simulink model "waypointFollower_Kohei"  (R2025a)
settings: Solver=ode23tb  StartTime=0.0  StopTime=130  FixedStep=.005  RelTol=1e-3  EnableMultiTasking=on
undefined symbols (not defined in the file): Cd, DiscIntNeverNeededParam, Kd_alt, Kd_p, Kd_q, Ki_alt, Ki_yaw, Kp_alt, Kp_p, Kp_pitch, Kp_pos, Kp_q, Kp_r, Kp_roll, Kp_vel, Kp_yaw, mass, mission, N_alt, N_p, N_q, rotorDir, rotorPositions, rotorThrustMax, rotorTimeConst, rotorTorqueMax, UAVsampleTime, x_area, y_area, z_area
libraries: simulink x9, slpidlib x9, uavalgslib x2, sim3dlib x2, uavsim3dlib x2, aerolibatmos2 x1, aerolibwind2 x1, shared6dof x1
(part 2 of 2)

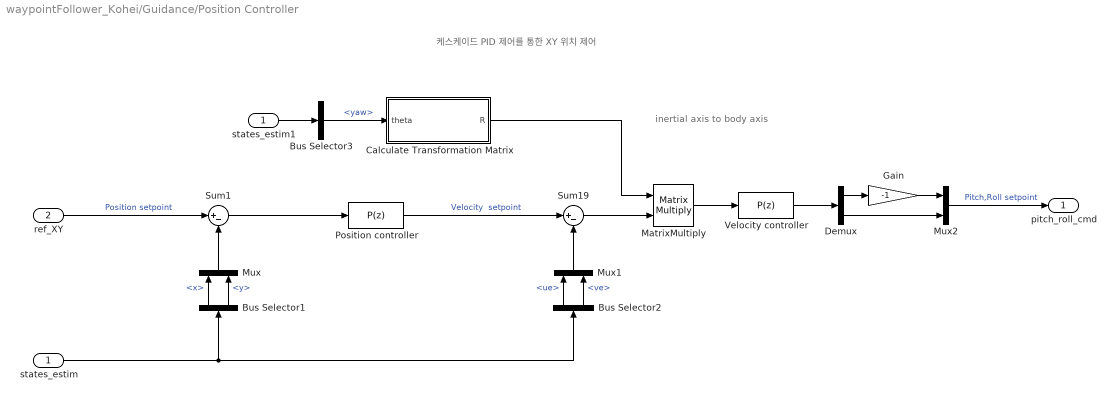
== system waypointFollower_Kohei/Guidance/Position Controller ==
  note: 케스케이드 PID 제어를 통한 XY 위치 제어
  note: inertial axis to body axis
  states_estim : Inport  OutDataTypeStr=Bus: UAVStateBUS
  ref_XY : Inport  Port=2
  Bus Selector1 : BusSelector  OutputSignals=x,y
  Bus Selector2 : BusSelector  OutputSignals=ue,ve
  Bus Selector3 : BusSelector  OutputSignals=yaw
  Calculate Transformation Matrix : Subsystem
  Demux : Demux  Outputs=2
  Gain : Gain  Gain=-1
  MatrixMultiply : Product  Multiplication=Matrix(*)
  Mux : Mux  Inputs=2
  Mux1 : Mux  Inputs=2
  Mux2 : Mux  Inputs=2
  Position controller : slpidlib/PID Controller  Controller=P  Form=Parallel  TimeDomain=Discrete-time  UseExternalTs=off  SampleTime=-1  IntegratorMethod=Forward Euler  FilterMethod=Forward Euler  ControllerParametersSource=internal  P=Kp_pos  I=0.1  UseKiTs=off  D=0  UseExternalDerivativeSource=off  N=100  UseFilter=on  TunerSelectOption=Transfer Function Based (PID Tuner App)  InitialConditionSource=internal  InitialConditionForIntegrator=0  InitialConditionForFilter=0  DifferentiatorICPrevScaledInput=0  ExternalReset=none  TrackingMode=off  Kt=1  LimitOutput=on  SatLimitsSource=internal  UpperSaturationLimit=4  LowerSaturationLimit=-4  LinearizeAsGain=on  AntiWindupMode=clamping  Kb=1  LimitIntegrator=off  UpperIntegratorSaturationLimit=inf  LowerIntegratorSaturationLimit=-inf  POutMin=[]  POutMax=[]  IOutMin=[]  IOutMax=[]  DOutMin=[]  DOutMax=[]  NOutMin=[]  NOutMax=[]  SumOutMin=[]  SumOutMax=[]  SaturationOutMin=[]  SaturationOutMax=[]  PParamMin=[]  PParamMax=[]  IParamMin=[]  IParamMax=[]  DParamMin=[]  DParamMax=[]  NParamMin=[]  NParamMax=[]  KbParamMin=[]  KbParamMax=[]  KtParamMin=[]  KtParamMax=[]  KbOutMin=[]  KbOutMax=[]  KtOutMin=[]  KtOutMax=[]  IntegratorOutMin=[]  IntegratorOutMax=[]  FilterOutMin=[]  FilterOutMax=[]  SumI1OutMin=[]  SumI1OutMax=[]  SumI2OutMin=[]  SumI2OutMax=[]  SumI3OutMin=[]  SumI3OutMax=[]  SumI4OutMin=[]  SumI4OutMax=[]  SumDOutMin=[]  SumDOutMax=[]  DifferentiatorOutMin=[]  DifferentiatorOutMax=[]  FilterDiffOutCoefMin=[]  FilterDiffOutCoefMax=[]  ReciprocalOutMin=[]  ReciprocalOutMax=[]  SumDenOutMin=[]  SumDenOutMax=[]  SumNumOutMin=[]  SumNumOutMax=[]  DivideOutMin=[]  DivideOutMax=[]  UdiffTsProdOutMin=[]  UdiffTsProdOutMax=[]  NTsProdOutMin=[]  NTsProdOutMax=[]  UintegralTsProdOutMin=[]  UintegralTsProdOutMax=[]  UngainTsProdOutMin=[]  UngainTsProdOutMax=[]  ClampingZeroOutDataTypeStr=Inherit: Inherit via back propagation  ClampingZeroOutMin=[]  ClampingZeroOutMax=[]  FilterDenConstantOutDataTypeStr=Inherit: Inherit via back propagation  FilterDenConstantOutMin=[]  FilterDenConstantOutMax=[]  PCopyOutDataTypeStr=Inherit: Inherit via back propagation  PCopyOutMin=[]  PCopyOutMax=[]  NCopyOutDataTypeStr=Inherit: Inherit via back propagation  NCopyOutMin=[]  NCopyOutMax=[]  IntegratorContinuousStateAttributes=''  IntegratorStateMustResolveToSignalObject=off  IntegratorRTWStateStorageClass=Auto  FilterContinuousStateAttributes=''  FilterStateMustResolveToSignalObject=off  FilterRTWStateStorageClass=Auto  ParallelPVariant=InternalParameters  IdealPVariant=Disabled  IVariant=Disabled  DVariant=Disabled  IntegratorVariant=Disabled  SatVariant=Enabled  AWVariant=Disabled  PCopyVariant=Disabled  TRVariant=Disabled  FdbkBlocksVariant=Forward  IdealPFdbkVariant=Disabled  SatFdbkVariant=Disabled  DerivativeFilterVariant=Disabled  NVariant=Disabled  NCopyVariant=Disabled_SignalSpec  FilterICVariant=Disabled  IntegratorICVariant=Disabled  ExternalResetVariant=Disabled  TRSumVariant=Passthrough  SumFdbkVariant=Disabled  SumVariant=Passthrough_P  TsampFilterVariant=InternalTs  TsampNgainVariant=Passthrough  TsampIntegralVariant=Disabled_SignalSpec  ExternalSaturationOutDataTypeStr=Inherit: Same as second input  DerivativeSourceVariant=Disabled  PreIntVariant=InternalPreInt
  Sum1 : Sum  Inputs=|+-
  Sum19 : Sum  Inputs=|+-
  Velocity controller : slpidlib/PID Controller  Controller=P  Form=Parallel  TimeDomain=Discrete-time  UseExternalTs=off  SampleTime=-1  IntegratorMethod=Forward Euler  FilterMethod=Forward Euler  ControllerParametersSource=internal  P=Kp_vel  I=0.075  UseKiTs=off  D=0  UseExternalDerivativeSource=off  N=100  UseFilter=on  TunerSelectOption=Transfer Function Based (PID Tuner App)  InitialConditionSource=internal  InitialConditionForIntegrator=0  InitialConditionForFilter=0  DifferentiatorICPrevScaledInput=0  ExternalReset=none  TrackingMode=off  Kt=1  LimitOutput=on  SatLimitsSource=internal  UpperSaturationLimit=20*pi/180  LowerSaturationLimit=-20*pi/180  LinearizeAsGain=on  AntiWindupMode=clamping  Kb=1  LimitIntegrator=off  UpperIntegratorSaturationLimit=inf  LowerIntegratorSaturationLimit=-inf  POutMin=[]  POutMax=[]  IOutMin=[]  IOutMax=[]  DOutMin=[]  DOutMax=[]  NOutMin=[]  NOutMax=[]  SumOutMin=[]  SumOutMax=[]  SaturationOutMin=[]  SaturationOutMax=[]  PParamMin=[]  PParamMax=[]  IParamMin=[]  IParamMax=[]  DParamMin=[]  DParamMax=[]  NParamMin=[]  NParamMax=[]  KbParamMin=[]  KbParamMax=[]  KtParamMin=[]  KtParamMax=[]  KbOutMin=[]  KbOutMax=[]  KtOutMin=[]  KtOutMax=[]  IntegratorOutMin=[]  IntegratorOutMax=[]  FilterOutMin=[]  FilterOutMax=[]  SumI1OutMin=[]  SumI1OutMax=[]  SumI2OutMin=[]  SumI2OutMax=[]  SumI3OutMin=[]  SumI3OutMax=[]  SumI4OutMin=[]  SumI4OutMax=[]  SumDOutMin=[]  SumDOutMax=[]  DifferentiatorOutMin=[]  DifferentiatorOutMax=[]  FilterDiffOutCoefMin=[]  FilterDiffOutCoefMax=[]  ReciprocalOutMin=[]  ReciprocalOutMax=[]  SumDenOutMin=[]  SumDenOutMax=[]  SumNumOutMin=[]  SumNumOutMax=[]  DivideOutMin=[]  DivideOutMax=[]  UdiffTsProdOutMin=[]  UdiffTsProdOutMax=[]  NTsProdOutMin=[]  NTsProdOutMax=[]  UintegralTsProdOutMin=[]  UintegralTsProdOutMax=[]  UngainTsProdOutMin=[]  UngainTsProdOutMax=[]  ClampingZeroOutDataTypeStr=Inherit: Inherit via back propagation  ClampingZeroOutMin=[]  ClampingZeroOutMax=[]  FilterDenConstantOutDataTypeStr=Inherit: Inherit via back propagation  FilterDenConstantOutMin=[]  FilterDenConstantOutMax=[]  PCopyOutDataTypeStr=Inherit: Inherit via back propagation  PCopyOutMin=[]  PCopyOutMax=[]  NCopyOutDataTypeStr=Inherit: Inherit via back propagation  NCopyOutMin=[]  NCopyOutMax=[]  IntegratorContinuousStateAttributes=''  IntegratorStateMustResolveToSignalObject=off  IntegratorRTWStateStorageClass=Auto  FilterContinuousStateAttributes=''  FilterStateMustResolveToSignalObject=off  FilterRTWStateStorageClass=Auto  ParallelPVariant=InternalParameters  IdealPVariant=Disabled  IVariant=Disabled  DVariant=Disabled  IntegratorVariant=Disabled  SatVariant=Enabled  AWVariant=Disabled  PCopyVariant=Disabled  TRVariant=Disabled  FdbkBlocksVariant=Forward  IdealPFdbkVariant=Disabled  SatFdbkVariant=Disabled  DerivativeFilterVariant=Disabled  NVariant=Disabled  NCopyVariant=Disabled_SignalSpec  FilterICVariant=Disabled  IntegratorICVariant=Disabled  ExternalResetVariant=Disabled  TRSumVariant=Passthrough  SumFdbkVariant=Disabled  SumVariant=Passthrough_P  TsampFilterVariant=InternalTs  TsampNgainVariant=Passthrough  TsampIntegralVariant=Disabled_SignalSpec  ExternalSaturationOutDataTypeStr=Inherit: Same as second input  DerivativeSourceVariant=Disabled  PreIntVariant=InternalPreInt
  states_estim1 : InportShadow  OutDataTypeStr=Bus: UAVStateBUS
  pitch_roll_cmd : Outport  VectorParamsAs1DForOutWhenUnconnected=off
  wires:
  ref_XY/1 -> Sum1/1  "Position setpoint"
  Sum1/1 -> Position controller/1
  Mux/1 -> Sum1/2
  Position controller/1 -> Sum19/1  "Velocity  setpoint"
  Velocity controller/1 -> Demux/1
  Mux2/1 -> pitch_roll_cmd/1  "Pitch,Roll setpoint"
  Bus Selector1/2 -> Mux/2  "<y>"
  Bus Selector1/1 -> Mux/1  "<x>"
  states_estim/1 -> Bus Selector2/1, Bus Selector1/1
  Bus Selector2/1 -> Mux1/1  "<ue>"
  Bus Selector2/2 -> Mux1/2  "<ve>"
  Mux1/1 -> Sum19/2
  Sum19/1 -> MatrixMultiply/2
  Calculate Transformation Matrix/1(R) -> MatrixMultiply/1
  MatrixMultiply/1 -> Velocity controller/1
  states_estim1/1 -> Bus Selector3/1
  Bus Selector3/1 -> Calculate Transformation Matrix/1(theta)  "<yaw>"
  Demux/1 -> Gain/1
  Gain/1 -> Mux2/1
  Demux/2 -> Mux2/2

== system waypointFollower_Kohei/Unreal/Subsystem ==
  In1 : Inport
  Bus Selector : BusSelector  OutputSignals=x,y,z
  Bus Selector1 : BusSelector  OutputSignals=yaw,pitch,roll
  Gain{,1..3} (4 alike) : Gain  Gain=-1
  Mux : Mux  Inputs=3
  Mux1 : Mux  Inputs=3
  Out1 : Outport
  Out2 : Outport  Port=2
  wires:
  In1/1 -> Bus Selector1/1, Bus Selector/1
  Gain1/1 -> Mux/3
  Bus Selector1/3 -> Mux1/3  "<roll>"
  Bus Selector/1 -> Mux/1  "<x>"
  Bus Selector1/2 -> Gain2/1  "<pitch>"
  Gain/1 -> Mux/2
  Bus Selector/2 -> Gain/1  "<y>"
  Gain2/1 -> Mux1/2
  Bus Selector1/1 -> Gain3/1  "<yaw>"
  Bus Selector/3 -> Gain1/1  "<z>"
  Mux1/1 -> Out2/1
  Mux/1 -> Out1/1
  Gain3/1 -> Mux1/1

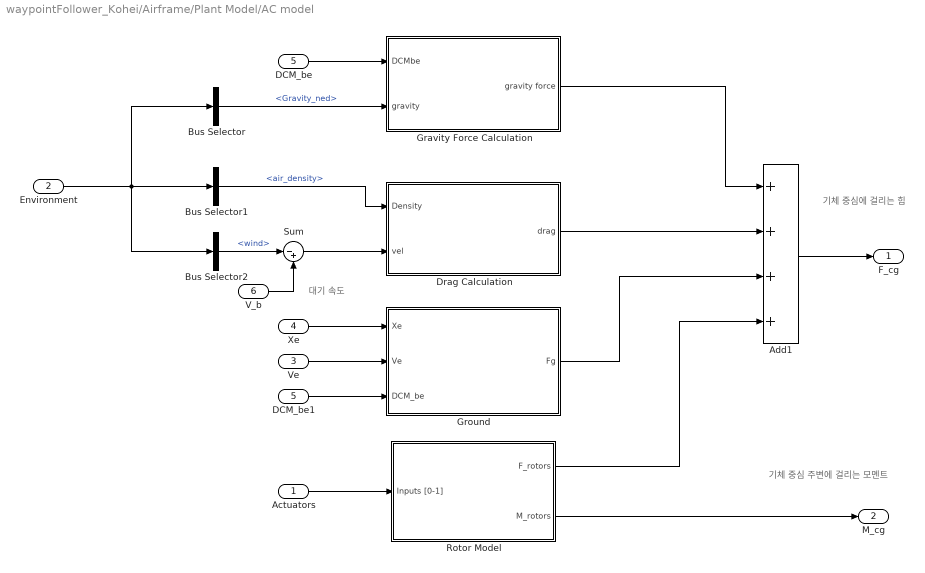
== system waypointFollower_Kohei/Airframe/Plant Model/AC model ==
  note: 기체 중심 주변에 걸리는 모멘트
  note: 기체 중심에 걸리는 힘
  note: 대기 속도
  Actuators : Inport
  Environment : Inport  Port=2
  Ve : Inport  Port=3
  Xe : Inport  Port=4
  DCM_be : Inport  Port=5
  V_b : Inport  Port=6  Unit=m/s
  Add1 : Sum  Inputs=++++
  Bus Selector : BusSelector  OutputSignals=Gravity_ned
  Bus Selector1 : BusSelector  OutputSignals=AtmosphereBus.air_density
  Bus Selector2 : BusSelector  OutputSignals=wind
  DCM_be1 : InportShadow  Port=5
  Drag Calculation : Subsystem
  Gravity Force Calculation : Subsystem
  Ground : Subsystem
  Rotor Model : Subsystem
  Sum : Sum  Inputs=|-+
  F_cg : Outport  Unit=N  VectorParamsAs1DForOutWhenUnconnected=off
  M_cg : Outport  Port=2  Unit=N*m  VectorParamsAs1DForOutWhenUnconnected=off
  wires:
  Add1/1 -> F_cg/1
  Rotor Model/2(M_rotors) -> M_cg/1
  Rotor Model/1(F_rotors) -> Add1/4
  Gravity Force Calculation/1(gravity force) -> Add1/1
  Environment/1 -> Bus Selector/1, Bus Selector2/1, Bus Selector1/1
  DCM_be/1 -> Gravity Force Calculation/1(DCMbe)
  Drag Calculation/1(drag) -> Add1/2
  Actuators/1 -> Rotor Model/1(Inputs [0-1])
  V_b/1 -> Sum/2
  Sum/1 -> Drag Calculation/2(vel)
  Bus Selector/1 -> Gravity Force Calculation/2(gravity)  "<Gravity_ned>"
  Bus Selector1/1 -> Drag Calculation/1(Density)  "<air_density>"
  Bus Selector2/1 -> Sum/1  "<wind>"
  Ground/1(Fg) -> Add1/3
  Xe/1 -> Ground/1(Xe)
  Ve/1 -> Ground/2(Ve)
  DCM_be1/1 -> Ground/3(DCM_be)

== system waypointFollower_Kohei/Airframe/Plant Model/Bus setup ==
  V_ned : Inport  Unit=m/second  PortDimensions=3
  X_ned : Inport  Port=2  Unit=m  PortDimensions=3
  Euler : Inport  Port=3  Unit=rad  PortDimensions=3
  Omega_b : Inport  Port=4  Unit=rad/s  PortDimensions=3
  Bus Creator : BusCreator  Inputs=12  OutDataTypeStr=Bus: UAVStateBUS  NonVirtualBus=on
  Demux{,1..3} (4 alike) : Demux  Outputs=3
  UAVState : Outport
  wires:
  Bus Creator/1 -> UAVState/1
  Demux/2 -> Bus Creator/2  "y"
  Demux3/2 -> Bus Creator/11  "q"
  Demux1/2 -> Bus Creator/5  "ve"
  Demux3/1 -> Bus Creator/10  "p"
  Demux/1 -> Bus Creator/1  "x"
  Demux2/3 -> Bus Creator/9  "yaw"
  Demux2/1 -> Bus Creator/7  "roll"
  Demux2/2 -> Bus Creator/8  "pitch"
  Demux3/3 -> Bus Creator/12  "r"
  Demux1/1 -> Bus Creator/4  "ue"
  Demux/3 -> Bus Creator/3  "z"
  X_ned/1 -> Demux/1
  Omega_b/1 -> Demux3/1
  Euler/1 -> Demux2/1
  V_ned/1 -> Demux1/1
  Demux1/3 -> Bus Creator/6  "we"

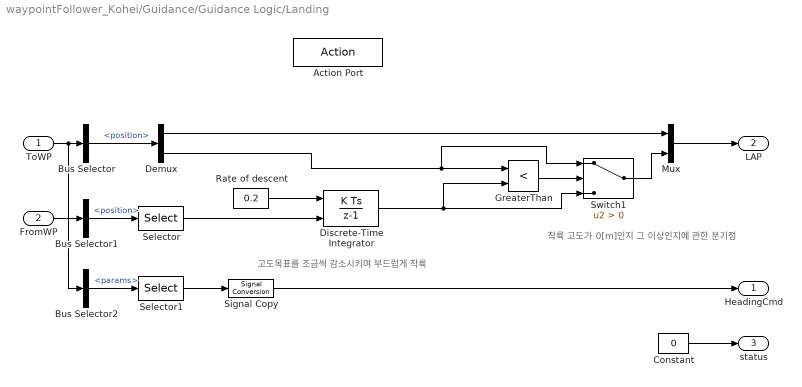
== system waypointFollower_Kohei/Guidance/Guidance Logic/Landing ==
  note: 착륙 고도가 0[m]인지 그 이상인지에 관한 분기점
  note: 고도목표를 조금씩 감소시키며 부드럽게 착륙
  ToWP : Inport
  FromWP : Inport  Port=2
  Action Port : ActionPort  ActionPortLabel=else
  Bus Selector : BusSelector  OutputSignals=position
  Bus Selector1 : BusSelector  OutputSignals=position
  Bus Selector2 : BusSelector  OutputSignals=params
  Constant : Constant  Value=0  OutDataTypeStr=boolean
  Demux : Demux  Outputs=[2 1]
  Discrete-Time Integrator : DiscreteIntegrator  InitialConditionSource=external  SampleTime=-1  LimitOutput=on  UpperSaturationLimit=0  ICPrevOutput=DiscIntNeverNeededParam  ICPrevScaledInput=DiscIntNeverNeededParam
  GreaterThan : RelationalOperator  Operator=<  OutDataTypeStr=boolean  RndMeth=Simplest  InputSameDT=off
  Mux : Mux  Inputs=2
  Rate of descent : Constant  Value=0.2
  Selector : Selector  InputPortWidth=3  IndexOptions=Index vector (dialog)  Indices=3  OutputSizes=1
  Selector1 : Selector  InputPortWidth=4  IndexOptions=Index vector (dialog)  Indices=1  OutputSizes=1
  Signal Copy : SignalConversion  OverrideOpt=off
  Switch1 : Switch  Criteria=u2 > Threshold  SaturateOnIntegerOverflow=off  InputSameDT=off
  HeadingCmd : Outport
  LAP : Outport  Port=2
  status : Outport  Port=3
  wires:
  Mux/1 -> LAP/1
  Constant/1 -> status/1
  Selector1/1 -> Signal Copy/1
  Bus Selector/1 -> Demux/1  "<position>"
  Demux/1 -> Mux/1
  FromWP/1 -> Bus Selector1/1
  Bus Selector1/1 -> Selector/1  "<position>"
  ToWP/1 -> Bus Selector2/1, Bus Selector/1
  Demux/2 -> Switch1/1, GreaterThan/1
  GreaterThan/1 -> Switch1/2
  Switch1/1 -> Mux/2
  Selector/1 -> Discrete-Time Integrator/2
  Rate of descent/1 -> Discrete-Time Integrator/1
  Discrete-Time Integrator/1 -> Switch1/3, GreaterThan/2
  Signal Copy/1 -> HeadingCmd/1
  Bus Selector2/1 -> Selector1/1  "<params>"

== system waypointFollower_Kohei/Guidance/Guidance Logic/Subsystem ==
  UAVState : Inport  OutDataTypeStr=Bus: UAVStateBUS
  Atan2 : Trigonometry  Operator=atan2
  Bus Selector1 : BusSelector  OutputSignals=x,y,z,ve,ue
  Mux : Mux
  Pose : Outport
  wires:
  Atan2/1 -> Mux/4  "course"
  UAVState/1 -> Bus Selector1/1
  Bus Selector1/1 -> Mux/1  "<x>"
  Bus Selector1/2 -> Mux/2  "<y>"
  Bus Selector1/3 -> Mux/3  "<z>"
  Mux/1 -> Pose/1
  Bus Selector1/4 -> Atan2/1  "<ve>"
  Bus Selector1/5 -> Atan2/2  "<ue>"

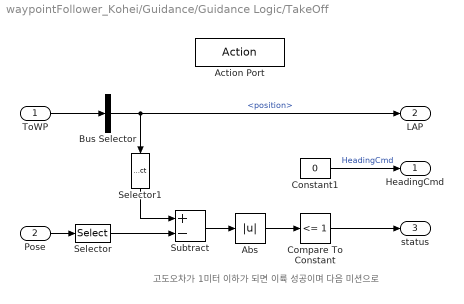
== system waypointFollower_Kohei/Guidance/Guidance Logic/TakeOff ==
  note: 고도오차가 1미터 이하가 되면 이륙 성공이며 다음 미션으로
  ToWP : Inport
  Pose : Inport  Port=2
  Action Port : ActionPort  ActionPortLabel=if(u1 == 1)
  Abs : Abs  SaturateOnIntegerOverflow=off
  Bus Selector : BusSelector  OutputSignals=position
  Compare To Constant : simulink/Logic and Bit Operations/Compare To Constant  relop=<=  const=1  OutDataTypeStr=boolean
  Constant1 : Constant  Value=0
  Selector : Selector  InputPortWidth=4  IndexOptions=Index vector (dialog)  Indices=3  OutputSizes=1
  Selector1 : Selector  InputPortWidth=3  IndexOptions=Index vector (dialog)  Indices=3  OutputSizes=1
  Subtract : Sum  Inputs=+-
  HeadingCmd : Outport
  LAP : Outport  Port=2
  status : Outport  Port=3
  wires:
  ToWP/1 -> Bus Selector/1
  Constant1/1 -> HeadingCmd/1  "HeadingCmd"
  Bus Selector/1 -> LAP/1, Selector1/1  "<position>"
  Pose/1 -> Selector/1
  Subtract/1 -> Abs/1
  Abs/1 -> Compare To Constant/1
  Compare To Constant/1 -> status/1
  Selector/1 -> Subtract/2
  Selector1/1 -> Subtract/1

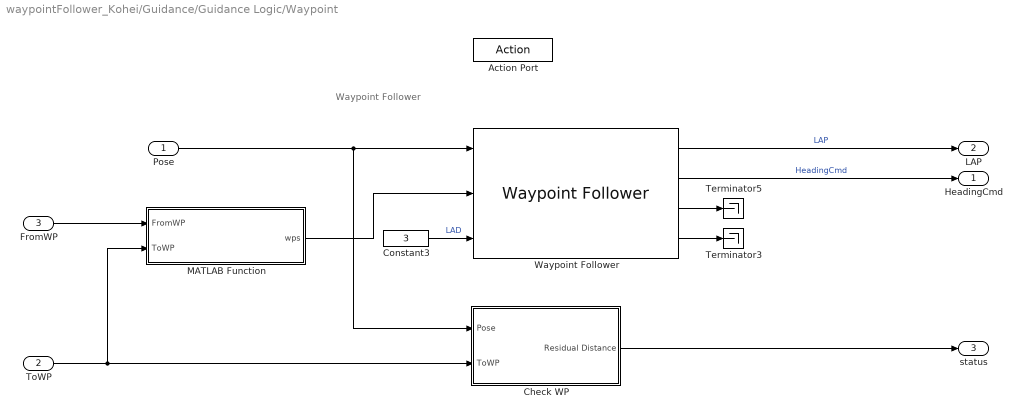
== system waypointFollower_Kohei/Guidance/Guidance Logic/Waypoint ==
  note: Waypoint Follower
  Pose : Inport
  ToWP : Inport  Port=2
  FromWP : Inport  Port=3
  Action Port : ActionPort  ActionPortLabel=elseif(u1 == 2)
  Check WP : Subsystem
  Constant3 : Constant  Value=3
  MATLAB Function : MATLAB Function  TreatAsAtomicUnit=on
  Terminator3 : Terminator
  Terminator5 : Terminator
  Waypoint Follower : uavalgslib/Waypoint Follower  UAVType=multirotor  StartFrom=first  TransitionRadiusSource=internal  TransitionRadius=10  MinLookaheadDistance=0.1  HoverAtLastWaypoint=off  YawInput=on  ShowCrossTrackErrorOutput=off  ShowStatusOutput=off  SimulateUsing=Interpreted execution
  HeadingCmd : Outport
  LAP : Outport  Port=2
  status : Outport  Port=3
  wires:
  Waypoint Follower/3 -> Terminator5/1
  ToWP/1 -> MATLAB Function/2(ToWP), Check WP/2(ToWP)
  Waypoint Follower/4 -> Terminator3/1
  Waypoint Follower/1 -> LAP/1  "LAP"
  MATLAB Function/1(wps) -> Waypoint Follower/2
  Constant3/1 -> Waypoint Follower/3  "LAD"
  Pose/1 -> Waypoint Follower/1, Check WP/1(Pose)
  FromWP/1 -> MATLAB Function/1(FromWP)
  Waypoint Follower/2 -> HeadingCmd/1  "HeadingCmd"
  Check WP/1(Residual Distance) -> status/1

== system waypointFollower_Kohei/Guidance/Position Controller/Calculate Transformation Matrix ==
  note: 피치 각도와 롤 각도는 작다고 가정하여 무시한 경우임 (즉, 꽤 평평하게 떠 다니는 드론)
  theta : Inport
  Gain : Gain  Gain=-1
  Matrix Concatenate : Concatenate  Mode=Multidimensional array
  Mux : Mux  Inputs=2
  Mux1 : Mux  Inputs=2
  Reshape : Reshape  OutputDimensionality=Row vector (2-D)
  Reshape1 : Reshape  OutputDimensionality=Row vector (2-D)
  SinCos : Trigonometry  Operator=sincos
  R : Outport
  wires:
  theta/1 -> SinCos/1
  SinCos/2 -> Mux1/2, Mux/1
  SinCos/1 -> Mux/2, Gain/1
  Mux/1 -> Reshape/1
  Mux1/1 -> Reshape1/1
  Matrix Concatenate/1 -> R/1
  Reshape/1 -> Matrix Concatenate/1
  Reshape1/1 -> Matrix Concatenate/2
  Gain/1 -> Mux1/1

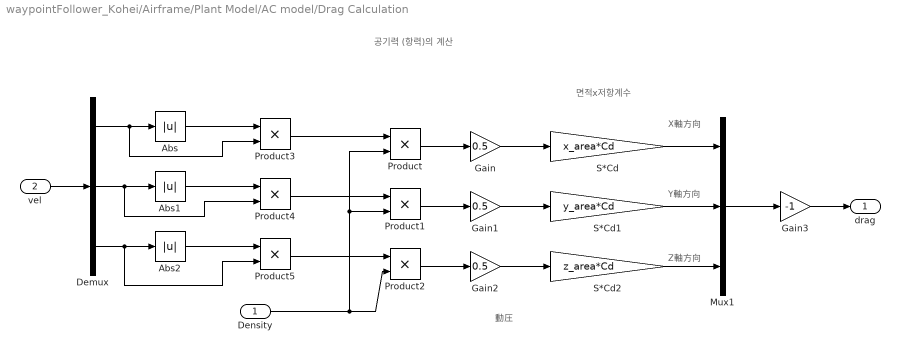
== system waypointFollower_Kohei/Airframe/Plant Model/AC model/Drag Calculation ==
  note: 動圧
  note: 면적x저항계수
  note: X軸方向
  note: 공기력 (항력)의 계산
  note: Y軸方向
  note: Z軸方向
  Density : Inport  Unit=kg/m^3
  vel : Inport  Port=2  Unit=m/s
  Abs : Abs  SaturateOnIntegerOverflow=off
  Abs1 : Abs  SaturateOnIntegerOverflow=off
  Abs2 : Abs  SaturateOnIntegerOverflow=off
  Demux : Demux  Outputs=3
  Gain : Gain  Gain=0.5
  Gain1 : Gain  Gain=0.5
  Gain2 : Gain  Gain=0.5
  Gain3 : Gain  Gain=-1
  Mux1 : Mux  Inputs=3
  Product{,1..5} (6 alike) : Product
  S*Cd : Gain  Gain=x_area*Cd
  S*Cd1 : Gain  Gain=y_area*Cd
  S*Cd2 : Gain  Gain=z_area*Cd
  drag : Outport  Unit=N  VectorParamsAs1DForOutWhenUnconnected=off
  wires:
  Gain3/1 -> drag/1
  Density/1 -> Product1/2, Product/2, Product2/2
  Product2/1 -> Gain2/1
  vel/1 -> Demux/1
  S*Cd/1 -> Mux1/1
  Abs/1 -> Product3/1
  Demux/3 -> Product5/2, Abs2/1
  Product/1 -> Gain/1
  Gain1/1 -> S*Cd1/1
  Abs2/1 -> Product5/1
  Product4/1 -> Product1/1
  Abs1/1 -> Product4/1
  Product1/1 -> Gain1/1
  Demux/1 -> Product3/2, Abs/1
  Gain/1 -> S*Cd/1
  Gain2/1 -> S*Cd2/1
  S*Cd1/1 -> Mux1/2
  Product5/1 -> Product2/1
  Product3/1 -> Product/1
  S*Cd2/1 -> Mux1/3
  Demux/2 -> Product4/2, Abs1/1
  Mux1/1 -> Gain3/1

== system waypointFollower_Kohei/Airframe/Plant Model/AC model/Gravity Force Calculation ==
  note: 기체의 축으로 변환
  note: 중력 계산
  DCMbe : Inport
  gravity : Inport  Port=2  Unit=m/s^2
  Gain1 : Gain  Gain=mass
  Product : Product  Multiplication=Matrix(*)
  gravity force : Outport  Unit=N  VectorParamsAs1DForOutWhenUnconnected=off
  wires:
  gravity/1 -> Gain1/1
  Gain1/1 -> Product/2  "gravity force NED"
  Product/1 -> gravity force/1
  DCMbe/1 -> Product/1

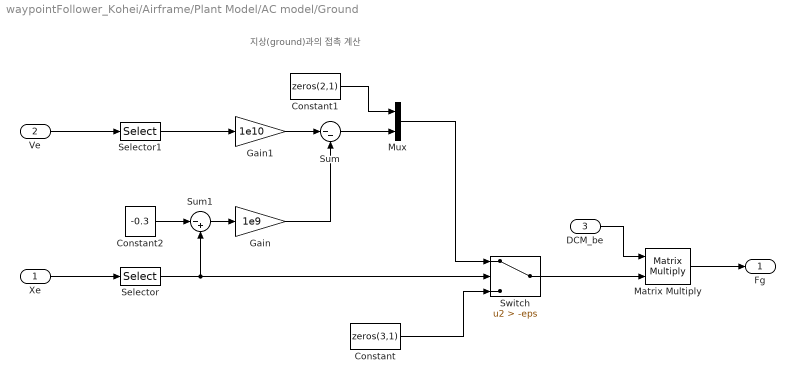
== system waypointFollower_Kohei/Airframe/Plant Model/AC model/Ground ==
  note: 지상(ground)과의 접촉 계산
  Xe : Inport
  Ve : Inport  Port=2
  DCM_be : Inport  Port=3
  Constant : Constant  Value=zeros(3,1)  VectorParams1D=off
  Constant1 : Constant  Value=zeros(2,1)  VectorParams1D=off
  Constant2 : Constant  Value=-0.3
  Gain : Gain  Gain=1e9
  Gain1 : Gain  Gain=1e10
  Matrix Multiply : Product  Multiplication=Matrix(*)
  Mux : Mux  Inputs=2
  Selector : Selector  InputPortWidth=3  IndexOptions=Index vector (dialog)  Indices=3  OutputSizes=1
  Selector1 : Selector  InputPortWidth=3  IndexOptions=Index vector (dialog)  Indices=3  OutputSizes=1
  Sum : Sum  Inputs=|--
  Sum1 : Sum  Inputs=|-+
  Switch : Switch  Criteria=u2 > Threshold  Threshold=-eps  SaturateOnIntegerOverflow=off  InputSameDT=off
  Fg : Outport
  wires:
  Xe/1 -> Selector/1
  Constant/1 -> Switch/3
  Ve/1 -> Selector1/1
  Gain/1 -> Sum/2
  Gain1/1 -> Sum/1
  Sum/1 -> Mux/2
  Mux/1 -> Switch/1
  Constant1/1 -> Mux/1
  Selector1/1 -> Gain1/1
  Selector/1 -> Sum1/2, Switch/2
  Sum1/1 -> Gain/1
  Constant2/1 -> Sum1/1
  Switch/1 -> Matrix Multiply/2
  DCM_be/1 -> Matrix Multiply/1
  Matrix Multiply/1 -> Fg/1

== system waypointFollower_Kohei/Airframe/Plant Model/AC model/Rotor Model ==
  note: 각 로터에서 발생하는 추력 또는 모멘트의 계산
      | ※각 다이나믹스를 단순한 1차 딜레이로 가정
  Inputs [0-1] : Inport
  Constant : Constant  Value=rotorPositions
  Constant1 : Constant  Value=rotorDir
  MATLAB Function : MATLAB Function  TreatAsAtomicUnit=on
  Thrust model : Subsystem
  Torque model : Subsystem
  F_rotors : Outport
  M_rotors : Outport  Port=2
  wires:
  Inputs [0-1]/1 -> Torque model/1(In1), Thrust model/1(In1)
  MATLAB Function/1(netF) -> F_rotors/1
  MATLAB Function/2(netM) -> M_rotors/1
  Constant/1 -> MATLAB Function/3(rotorPositions)
  Constant1/1 -> MATLAB Function/4(rotorDir)
  Torque model/1(Out1) -> MATLAB Function/2(tauEachRotor)
  Thrust model/1(Out1) -> MATLAB Function/1(thrustEachRotor)

== system waypointFollower_Kohei/Guidance/Guidance Logic/Waypoint/Check WP ==
  note: 각 축의 위치가 목표지점을 일정 범위를 통과했다면 다음 미션으로
  Pose : Inport
  ToWP : Inport  Port=2
  Abs : Abs  SaturateOnIntegerOverflow=off
  Bus Selector : BusSelector  OutputSignals=position
  Compare To Constant : simulink/Logic and Bit Operations/Compare To Constant  relop=<=  const=5  OutDataTypeStr=boolean
  Compare To Constant1 : simulink/Logic and Bit Operations/Compare To Constant  relop===  const=3  OutDataTypeStr=boolean
  Demux : Demux  Outputs=[3 1]
  Sum : Sum  Inputs=-+
  Sum of Elements : Sum  Inputs=+
  Terminator : Terminator
  Residual Distance : Outport
  wires:
  Demux/2 -> Terminator/1
  Demux/1 -> Sum/1
  Pose/1 -> Demux/1
  ToWP/1 -> Bus Selector/1
  Bus Selector/1 -> Sum/2  "<position>"
  Sum/1 -> Abs/1
  Abs/1 -> Compare To Constant/1
  Compare To Constant/1 -> Sum of Elements/1
  Sum of Elements/1 -> Compare To Constant1/1
  Compare To Constant1/1 -> Residual Distance/1

== system waypointFollower_Kohei/Airframe/Plant Model/AC model/Rotor Model/Thrust model ==
  In1 : Inport
  Demux : Demux
  Mux : Mux
  Transfer Fcn{,2..4} (4 alike) : TransferFcn  Numerator=[rotorThrustMax]  Denominator=[rotorTimeConst 1]
  Out1 : Outport
  wires:
  Transfer Fcn3/1 -> Mux/2
  Demux/1 -> Transfer Fcn4/1
  Transfer Fcn2/1 -> Mux/3
  Demux/3 -> Transfer Fcn2/1
  Mux/1 -> Out1/1
  Transfer Fcn4/1 -> Mux/1
  Demux/4 -> Transfer Fcn/1
  Demux/2 -> Transfer Fcn3/1
  Transfer Fcn/1 -> Mux/4
  In1/1 -> Demux/1

== system waypointFollower_Kohei/Airframe/Plant Model/AC model/Rotor Model/Torque model ==
  In1 : Inport
  Demux : Demux
  Mux : Mux
  Transfer Fcn{1..4} (4 alike) : TransferFcn  Numerator=[rotorTorqueMax]  Denominator=[rotorTimeConst 1]
  Out1 : Outport
  wires:
  Transfer Fcn4/1 -> Mux/4
  Demux/1 -> Transfer Fcn1/1
  Transfer Fcn3/1 -> Mux/3
  Transfer Fcn2/1 -> Mux/2
  Demux/2 -> Transfer Fcn2/1
  Demux/4 -> Transfer Fcn4/1
  Demux/3 -> Transfer Fcn3/1
  Mux/1 -> Out1/1
  Transfer Fcn1/1 -> Mux/1
  In1/1 -> Demux/1

== matlab function waypointFollower_Kohei/Control/Yaw Controller/MATLAB Function1 ==
  data: u input; y output
function y = wrapYaw(u)
if (u>pi)
    y = u - 2*pi;
elseif(u<-pi)
    y = u + 2*pi;
else
    y=u;
end

== matlab function waypointFollower_Kohei/Guidance/Guidance Logic/Waypoint/MATLAB Function ==
  data: FromWP input; wps output; ToWP input
function wps = getWaypointMission(FromWP, ToWP)

persistent outWPS

if isempty(outWPS)
    outWPS = zeros(2,4);
end

outWPS(1,:) = [FromWP.position' FromWP.params(1)];
outWPS(2,:) = [ToWP.position' ToWP.params(1)];

wps = outWPS;

== matlab function waypointFollower_Kohei/Control/Yaw Controller/MATLAB Function ==
  data: u input; y output
function y = wrapYaw(u)
if (u>pi)
    y = u - 2*pi;
elseif(u<-pi)
    y = u + 2*pi;
else
    y=u;
end

== matlab function waypointFollower_Kohei/Airframe/Plant Model/AC model/Rotor Model/MATLAB Function ==
  data: thrustEachRotor input; tauEachRotor input; rotorPositions input; netF output; netM output; rotorDir input
function [netF, netM] = getForceMoment(thrustEachRotor, tauEachRotor, rotorPositions, rotorDir)
%#codegen
Fx = 0;
Fy = 0;
Fz = -sum(thrustEachRotor);

netF = [Fx; Fy; Fz];

netM = [0; 0; 0]; %initialize
    for i = 1:4
        rotPos = rotorPositions(:, i);
        Fi = [0, 0, -thrustEachRotor(i)]';
        netM = netM +  cross(rotPos, Fi);%contribution from thrusts of each propeller
        netM(3) = netM(3) - rotorDir(i)*tauEachRotor(i); %contribution from counter torque acting on propeller
    end

end
